simulink model "Simulacija_21a"  (R2021a)
settings: Solver=ode23t  StartTime=0.0  StopTime=10  MaxStep=1e-4  RelTol=1e-5
values from neighbouring files (symbols this model uses):
  J = 0.5    [Inicijalizacija_22.m]
  Kpi = 0.2    [Inicijalizacija_22.m]
  Kpw = 10/150    (= 0.0666666666667)    [Inicijalizacija_22.m]
  La = 0.025    [Inicijalizacija_22.m]
  mn = PsiFn*In    (= 35.8706304467)    [Inicijalizacija_22.m]
  PsiFn = (Un-Ra*In)/wn    (= 1.37963963256)    [Inicijalizacija_22.m]
  Ra = 0.9    [Inicijalizacija_22.m]
  Ts = 10e-6    (= 1e-05)    [Inicijalizacija_22.m]
  Udc = 250    [Inicijalizacija_22.m]
  wn = nn*pi/30    (= 149.749249821)    [Inicijalizacija_22.m]
libraries: spsDCMachineLib x1, spsFullBridgeConverterLib x1, spsPWMGenerator2LevelLib x1, spsVoltageMeasurementLib x1, spsCurrentMeasurementLib x1, spsDCVoltageSourceLib x1, spspowerguiLib x1
settings Model: Creator=Milan  LastModifiedBy=Nikola
settings SolverCC: ZeroCrossAlgorithm=Adaptive  AlgebraicLoopSolver=TrustRegion
settings DataIOCC: SaveFormat=StructureWithTime  ReturnWorkspaceOutputs=off
settings OptimizationCC: LifeSpan=inf
settings DebuggingCC: SFExecutionAtInitializationDiag=none  SFMachineParentedDataDiag=warning  ArithmeticOperatorsInVariantConditions=warning
settings HardwareCC: ProdBitPerSizeT=32  ProdBitPerPtrDiffT=32  ProdWordSize=32  ProdHWDeviceType=Specified
settings SFSimCC: SimUseLocalCustomCode=off  CustomCodeUndefinedFunction=UseInterfaceOnly
settings RTWCC: RTWUseLocalCustomCode=off
settings CodeAppCC: StateflowObjectComments=on
settings SimscapeCC: SimscapeNormalizeSystem=off

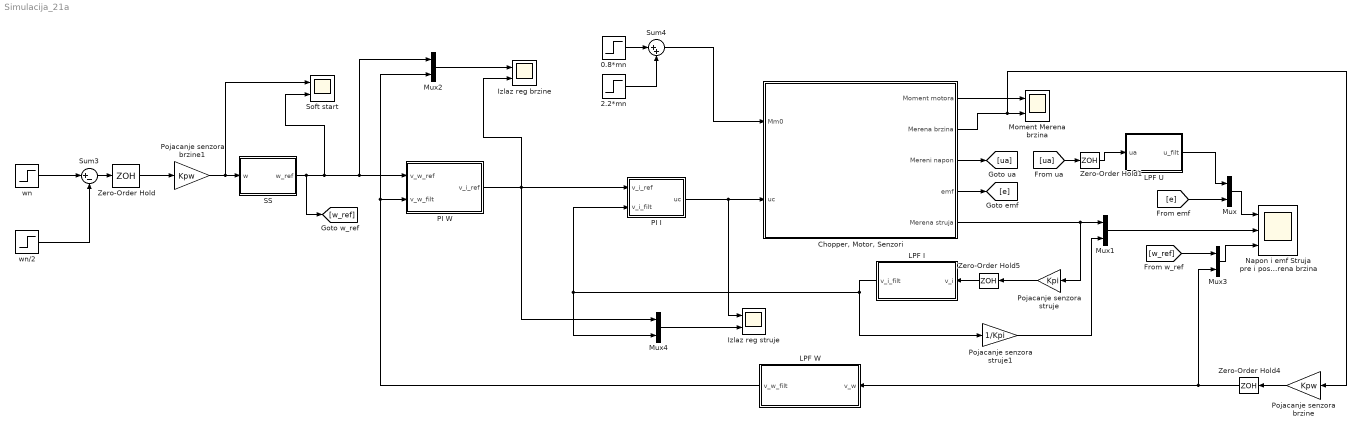
== system Simulacija_21a ==
  0.8*mn : Step  Time=3.5  After=0.8*mn  SampleTime=0
  2.2*mn : Step  Time=6.5  After=2.2*mn  SampleTime=0
  "Chopper, Motor, Senzori" : Subsystem
  Izlaz reg brzine : Scope  NumInputPorts=2
  Izlaz reg struje : Scope  NumInputPorts=2
  LPF I : MATLAB Function  TreatAsAtomicUnit=on
  LPF U : MATLAB Function  TreatAsAtomicUnit=on
  LPF W : MATLAB Function  TreatAsAtomicUnit=on
  Moment Merena brzina : Scope  NumInputPorts=2
  Mux{,1..4} (5 alike) : Mux  Inputs=2
  Napon i emf Struja pre i posle filtera Referentna i merena brzina : Scope  NumInputPorts=3
  PI I : MATLAB Function  TreatAsAtomicUnit=on
  PI W : MATLAB Function  TreatAsAtomicUnit=on
  Pojacanje senzora brzine : Gain  Gain=Kpw
  Pojacanje senzora brzine1 : Gain  Gain=Kpw
  Pojacanje senzora struje : Gain  Gain=Kpi
  Pojacanje senzora struje1 : Gain  Gain=1/Kpi
  SS : MATLAB Function  TreatAsAtomicUnit=on
  Soft start : Scope  NumInputPorts=2
  Sum3 : Sum  Inputs=|+-
  Sum4 : Sum  Inputs=|++
  Zero-Order Hold{,1,4..5} (4 alike) : ZeroOrderHold  SampleTime=Ts
  wn : Step  Time=0.1  After=wn  SampleTime=0
  "wn/2 " : Step  Time=4.5  After=wn/2  SampleTime=0
  wires:
  Mux/1 -> Napon i emf Struja pre i posle filtera Referentna i merena brzina/1
  Mux1/1 -> Napon i emf Struja pre i posle filtera Referentna i merena brzina/2
  [e] -> Mux/2
  "Chopper, Motor, Senzori"/3(Mereni napon) -> [ua]
  LPF U/1(u_filt) -> Mux/1
  Mux3/1 -> Napon i emf Struja pre i posle filtera Referentna i merena brzina/3
  "Chopper, Motor, Senzori"/1(Moment motora) -> Moment Merena brzina/1
  "Chopper, Motor, Senzori"/4(emf) -> [e]
  "Chopper, Motor, Senzori"/5(Merena struja) -> Mux1/1, Pojacanje senzora struje/1
  [w_ref] -> Mux3/1
  "Chopper, Motor, Senzori"/2(Merena brzina) -> Pojacanje senzora brzine/1, Moment Merena brzina/2
  Mux2/1 -> Izlaz reg brzine/1
  0.8*mn/1 -> Sum4/1
  "wn/2 "/1 -> Sum3/2
  Sum4/1 -> "Chopper, Motor, Senzori"/1(Mm0)
  Mux4/1 -> Izlaz reg struje/2
  2.2*mn/1 -> Sum4/2
  PI I/1(uc) -> Izlaz reg struje/1, "Chopper, Motor, Senzori"/2(uc)
  wn/1 -> Sum3/1
  LPF W/1(v_w_filt) -> Mux2/2, PI W/2(v_w_filt)
  Sum3/1 -> Zero-Order Hold/1
  PI W/1(v_i_ref) -> Mux4/1, Izlaz reg brzine/2, PI I/1(v_i_ref)
  LPF I/1(v_i_filt) -> Pojacanje senzora struje1/1, PI I/2(v_i_filt), Mux4/2
  [ua] -> Zero-Order Hold1/1
  Zero-Order Hold1/1 -> LPF U/1(ua)
  Zero-Order Hold5/1 -> LPF I/1(v_i)
  Pojacanje senzora struje1/1 -> Mux1/2
  Zero-Order Hold4/1 -> Mux3/2, LPF W/1(v_w)
  Zero-Order Hold/1 -> Pojacanje senzora brzine1/1
  Pojacanje senzora brzine1/1 -> Soft start/1, SS/1(w)
  SS/1(w_ref) -> [w_ref], Soft start/2, PI W/1(v_w_ref), Mux2/1
  Pojacanje senzora brzine/1 -> Zero-Order Hold4/1
  Pojacanje senzora struje/1 -> Zero-Order Hold5/1

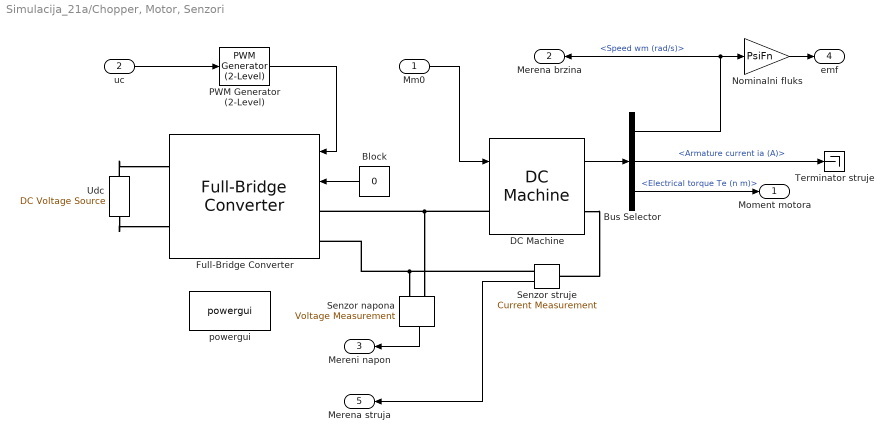
== system Simulacija_21a/Chopper, Motor, Senzori ==
  Mm0 : Inport
  uc : Inport  Port=2
  Block : Constant  Value=0
  Bus Selector : BusSelector  OutputSignals=Speed wm (rad/s),Armature current ia (A),Electrical torque Te (n m)
  DC Machine : spsDCMachineLib/DC Machine  PresetModel=No  MechanicalLoad=Torque TL  FieldType=Permanent magnet  ShowDetailedParameters=on  MeasurementBus=off  RLa="[ Ra  La]"  RLf="[ 240  120]"  Laf=1.8  MachineConstant=Torque constant (N.m/A)  Ke=1.8  Kt=PsiFn  J=J  Bm=0  Tf=0  w0=0  Ifinit=1  TsPowergui=0  TsBlock=-1
  Full-Bridge Converter : spsFullBridgeConverterLib/Full-Bridge Converter  ModelType=Switching devices  Ron=1e-3  Rs=1e6  Cs=inf  Vforward=[0,0]  Ron_Diode=1e-3  Rs_Diode=1e6  Cs_Diode=inf  Vf_Diode=1e-3  Rs_CurrentSource=inf
      settings: SourceProductBaseCode=PS
  Nominalni fluks : Gain  Gain=PsiFn
  PWM Generator (2-Level) : spsPWMGenerator2LevelLib/PWM Generator (2-Level)  ModulatorType=Single-phase full-bridge (4 pulses)  ModulatorMode=Unsynchronized  Fc=fc  Pc=90  nF=27  MinMax="[ -1  1 ]"  SamplingTechnique=Natural  ModulatingSignals=off  m=0.8  Freq=60  Phase=0  Ts=0  ShowCarrierOutport=off
  Senzor napona : spsVoltageMeasurementLib/Voltage Measurement  PhasorSimulation=off  OutputType=Complex  PSBequivalent=0
  Senzor struje : spsCurrentMeasurementLib/Current Measurement  PhasorSimulation=off  OutputType=Complex  PSBequivalent=0
  Terminator struje : Terminator
  Udc : spsDCVoltageSourceLib/DC Voltage Source  Amplitude=Udc  Measurements=None
  powergui : spspowerguiLib/powergui  Priority=1  SimulationMode=Continuous  SampleTime=50e-6  frequency=60  Iterations=50  frequencyindice=0  Pbase=100e6  ErrMax=1e-4  UnitsV=kV  UnitsW=MW  buscounter=0  FunctionMessages=off  echomessages=off  EnableUseOfTLC=off  CurrentSourceSwitches=off  DisableSnubberDevices=off  DisableRonSwitches=off  DisableVfSwitches=off  DisplayEquations=off  AutomaticDiscreteSolvers=off  SolverType=Tustin/Backward Euler (TBE)  Interpol=off  ExternalGateDelay=off  methode=off  Ts=100  x0status=blocks  SPID=on  SwTol=0  HookPort=off  NonlinearTolerance=1e-4  nMaxIteration=100  ContinueOnMaxIteration=off  RestoreLinks=warning  ResistiveCurrentMeasurement=off  Frange=[0:2:500]  Ylog=off  Xlog=on  ShowGrid=off  save=off  variable=ZData  structure=0  ZoomFFT=off  StartTime=0.0  cycles=1  DisplayStyle=1  fundamental=60  FreqAxis=off  MaxFrequency=1000  frequencyindicesteady=1  RmsSteady=1  display=off
  Moment motora : Outport
  Merena brzina : Outport  Port=2
  Mereni napon : Outport  Port=3
  emf : Outport  Port=4
  Merena struja : Outport  Port=5
  wires:
  Senzor napona/1 -> Mereni napon/1
  uc/1 -> PWM Generator (2-Level)/1
  Block/1 -> Full-Bridge Converter/2
  Mm0/1 -> DC Machine/1
  PWM Generator (2-Level)/1 -> Full-Bridge Converter/1
  DC Machine/1 -> Bus Selector/1
  Senzor struje/1 -> Merena struja/1
  Bus Selector/3 -> Moment motora/1  "<Electrical torque Te (n m)>"
  Bus Selector/2 -> Terminator struje/1  "<Armature current ia (A)>"
  Bus Selector/1 -> Merena brzina/1, Nominalni fluks/1  "<Speed wm (rad/s)>"
  Nominalni fluks/1 -> emf/1
  connections:
  DC Machine/LConn1 -- Full-Bridge Converter/LConn1 -- Senzor napona/LConn1
  Senzor struje/RConn1 -- Full-Bridge Converter/LConn2 -- Senzor napona/LConn2
  DC Machine/RConn1 -- Senzor struje/LConn1
  Udc/LConn1 -- Full-Bridge Converter/RConn2
  Udc/RConn1 -- Full-Bridge Converter/RConn1

== matlab function Simulacija_21a/SS ==
  data: w input; w_ref output
function w_ref = soft_start(w)

%% Podaci
Ts=10e-6;

%% Soft-start

return

== matlab function Simulacija_21a/PI W ==
  data: v_w_ref input; v_w_filt input; v_i_ref output
function v_i_ref = PI(v_w_ref,v_w_filt)

%% Podaci
Ts=10e-6;

%% PI
       
return

== matlab function Simulacija_21a/LPF I ==
  data: v_i input; v_i_filt output
    function v_i_filt = LPF(v_i)

%% Podaci
Ts=10e-6;

%% LPF

return

== matlab function Simulacija_21a/PI I ==
  data: v_i_ref input; v_i_filt input; uc output
function uc = PI(v_i_ref,v_i_filt)

%% Podaci
Ts=10e-6;

%% PI

return

== matlab function Simulacija_21a/LPF U ==
  data: ua input; u_filt output
    function u_filt = LPF(ua)

%% Podaci
Ts=10e-6;

%% LPF

return

== matlab function Simulacija_21a/LPF W ==
  data: v_w input; v_w_filt output
    function v_w_filt = LPF(v_w)

%% Podaci
Ts=10e-6;

%% LPF

return
